simulink model "SpaceVectorPWM"  (R2018a)
settings: Solver=FixedStepDiscrete  StartTime=0.0  StopTime=0.2  FixedStep=1e-5  RelTol=1e-3
values from neighbouring files (symbols this model uses):
  A = 1    [SpaceVector.m]
  f_c = 5e4    (= 50000)    [PWM.m]    (also in SpaceVector.m = 50; SpwmTpwm.m = 50)
  f_s = 10000    [SpaceVector.m]    (also in SpaceVectorOnlyCode.m = 1000; SpwmTpwm.m)
undefined symbols (not defined in the file or in its folder): Vdc
libraries: simulink_extras x1, powerlib_meascontrol x1, simulink x1
settings Model: Creator=enes_  LastModifiedBy=enes_

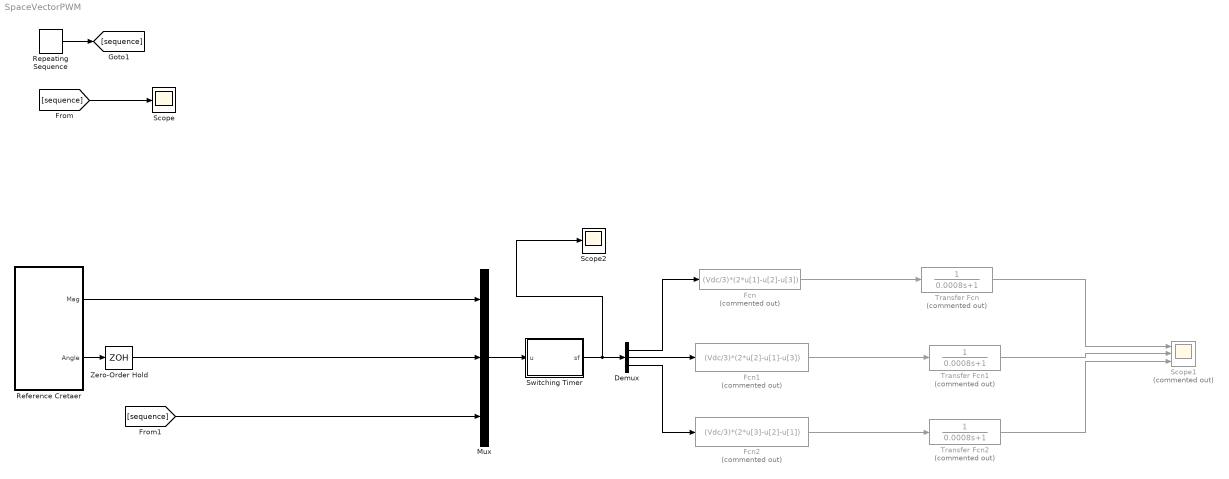
== system SpaceVectorPWM ==
  Demux : Demux  Outputs=3
  Fcn : Fcn  Commented=on  Expr=(Vdc/3)*(2*u[1]-u[2]-u[3])
  Fcn1 : Fcn  Commented=on  Expr=(Vdc/3)*(2*u[2]-u[1]-u[3])
  Fcn2 : Fcn  Commented=on  Expr=(Vdc/3)*(2*u[3]-u[2]-u[1])
  Mux : Mux  Inputs=3
  Reference Cretaer : Subsystem
  Repeating Sequence : simulink/Sources/Repeating Sequence  rep_seq_t=[0 1 2 3 4] /f_s  rep_seq_y=[-1 0 1 0 -1]
  Scope : Scope
  Scope1 : Scope  Commented=on  NumInputPorts=3
  Scope2 : Scope
  Switching Timer : MATLAB Function  TreatAsAtomicUnit=on
  Transfer Fcn : TransferFcn  Commented=on  Denominator=[0.0008 1]
  Transfer Fcn1 : TransferFcn  Commented=on  Denominator=[0.0008 1]
  Transfer Fcn2 : TransferFcn  Commented=on  Denominator=[0.0008 1]
  Zero-Order Hold : ZeroOrderHold  SampleTime=-1
  wires:
  [sequence] -> Scope/1
  Repeating Sequence/1 -> [sequence]
  Reference Cretaer/1("Mag ") -> Mux/1
  [sequence] -> Mux/3
  Reference Cretaer/2(Angle) -> Zero-Order Hold/1
  Zero-Order Hold/1 -> Mux/2
  Mux/1 -> Switching Timer/1(u)
  Switching Timer/1(sf) -> Demux/1, Scope2/1
  Fcn2/1 -> Transfer Fcn2/1
  Fcn1/1 -> Transfer Fcn1/1
  Fcn/1 -> Transfer Fcn/1
  Transfer Fcn/1 -> Scope1/1
  Transfer Fcn1/1 -> Scope1/2
  Transfer Fcn2/1 -> Scope1/3
  Demux/1 -> Fcn/1
  Demux/2 -> Fcn1/1
  Demux/3 -> Fcn2/1

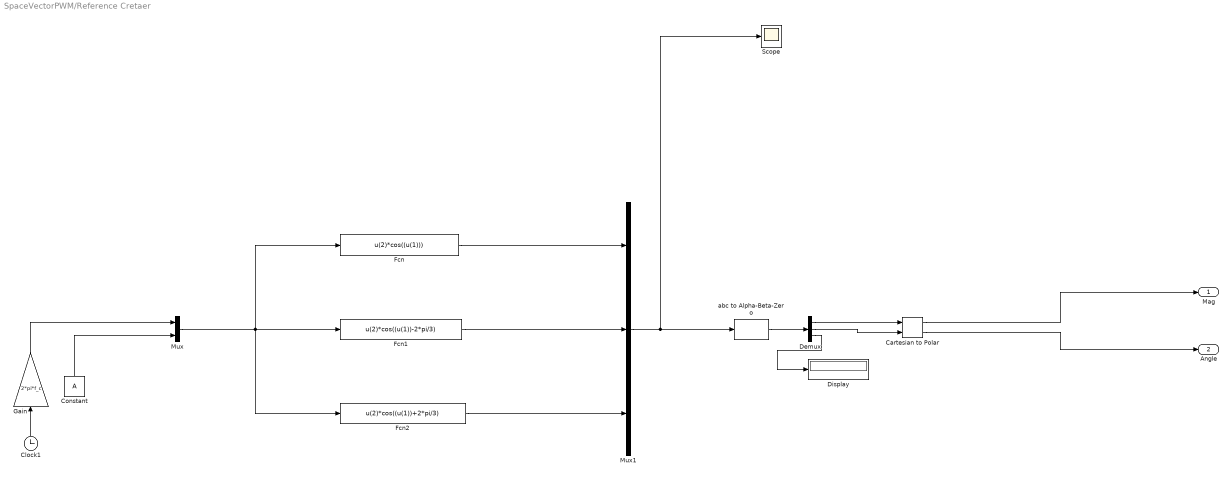
== system SpaceVectorPWM/Reference Cretaer ==
  Cartesian to Polar : simulink_extras/Transformations/Cartesian to Polar
      settings: SourceProductName=Simulink
  Clock1 : Clock
  Constant : Constant  Value=A
  Demux : Demux  Outputs=3
  Display : Display
  Fcn : Fcn  Expr=u(2)*cos((u(1)))
  Fcn1 : Fcn  Expr=u(2)*cos((u(1))-2*pi/3)
  Fcn2 : Fcn  Expr=u(2)*cos((u(1))+2*pi/3)
  Gain : Gain  Gain=2*pi*f_c
  Mux : Mux  Inputs=2
  Mux1 : Mux  Inputs=3
  Scope : Scope
  abc to Alpha-Beta-Zero : powerlib_meascontrol/Transformations/abc to Alpha-Beta-Zero
      settings: SourceProductName=Simscape Power Systems
  "Mag " : Outport
  Angle : Outport  Port=2
  wires:
  Mux/1 -> Fcn2/1, Fcn1/1, Fcn/1
  Constant/1 -> Mux/2
  Gain/1 -> Mux/1
  Mux1/1 -> abc to Alpha-Beta-Zero/1, Scope/1
  Fcn2/1 -> Mux1/3
  Fcn/1 -> Mux1/1
  Clock1/1 -> Gain/1
  Fcn1/1 -> Mux1/2
  abc to Alpha-Beta-Zero/1 -> Demux/1
  Demux/1 -> Cartesian to Polar/1
  Demux/2 -> Cartesian to Polar/2
  Cartesian to Polar/1 -> "Mag "/1
  Cartesian to Polar/2 -> Angle/1
  Demux/3 -> Display/1

== matlab function SpaceVectorPWM/Switching Timer ==
  data: u input; sf output
%Matlab Code to generate Switching functions
% Inputs are magnitude u1(:),angle u2(:)
% and ramp time signal for comparison u3(:)
function sf =SwitchingTimer(u)
ts=0.0002;vdc=1;peak_phase_max= vdc/sqrt(3);
x=u(2); y=u(3); mag=(u(1)/peak_phase_max) * ts;
%sector I
 if (x>=0) & (x<pi/3)
 ta = mag * sin(pi/3-x);tb = mag * sin(x);
 t0 =(ts-ta-tb);
t1=[t0/4 ta/2 tb/2 t0/2 tb/2 ta/2 t0/4];t1=cumsum(t1);
v1=[0 1 1 1 1 1 0];v2=[0 0 1 1 1 0 0];v3=[0 0 0 1 0 0 0];
 for j=1:7
 if(y<t1(j))
 break
 end
 end
 sa=v1(j);sb=v2(j);sc=v3(j);
end
% sector II
 if (x>=pi/3) & (x<2*pi/3)
 adv= x-pi/3;
tb = mag * sin(pi/3-adv);ta = mag * sin(adv);
t0 =(ts-ta-tb);
t1=[t0/4 ta/2 tb/2 t0/2 tb/2 ta/2 t0/4];t1=cumsum(t1);
v1=[0 0 1 1 1 0 0];v2=[0 1 1 1 1 1 0];v3=[0 0 0 1 0 0 0];
 for j=1:7
 if(y<t1(j))
 break
 end
 end
 sa=v1(j);sb=v2(j);sc=v3(j);
 end
%sector III
 if (x>=2*pi/3) & (x<pi)
 adv=x-2*pi/3;
ta = mag * sin(pi/3-adv);tb = mag * sin(adv);
 t0 =(ts-ta-tb);
t1=[t0/4 ta/2 tb/2 t0/2 tb/2 ta/2 t0/4];t1=cumsum(t1);
v1=[0 0 0 1 0 0 0];v2=[0 1 1 1 1 1 0];v3=[0 0 1 1 1 0 0];
 for j=1:7
 if(y<t1(j))
 break
 end
 end
 sa=v1(j);sb=v2(j);sc=v3(j);
end
%sector IV
 if (x>=-pi) & (x<-2*pi/3)
 adv = x + pi;
tb= mag * sin(pi/3 - adv);ta = mag * sin(adv);
 t0 =(ts-ta-tb);
t1=[t0/4 ta/2 tb/2 t0/2 tb/2 ta/2 t0/4];t1=cumsum(t1);
v1=[0 0 0 1 0 0 0];v2=[0 0 1 1 1 0 0];v3=[0 1 1 1 1 1 0];
 for j=1:7
 if(y<t1(j))
 break
 end
 end
 sa=v1(j);sb=v2(j);sc=v3(j);
end
% sector V
 if (x>=-2*pi/3) & (x<-pi/3)
 adv = x+2*pi/3;
ta = mag * sin(pi/3-adv);tb = mag * sin(adv);
 t0 =(ts-ta-tb);
t1=[t0/4 ta/2 tb/2 t0/2 tb/2 ta/2 t0/4];t1=cumsum(t1);
v1=[0 0 1 1 1 0 0];v2=[0 0 0 1 0 0 0];v3=[0 1 1 1 1 1 0];
 for j=1:7
 if(y<t1(j))
 break
 end
 end
 sa=v1(j);sb=v2(j);sc=v3(j);
end
%Sector VI
 if (x>=-pi/3) & (x<0)
 adv = x+pi/3;
tb = mag * sin(pi/3-adv);ta = mag * sin(adv);
 t0 =(ts-ta-tb);
t1=[t0/4 ta/2 tb/2 t0/2 tb/2 ta/2 t0/4];t1=cumsum(t1);
v1=[0 1 1 1 1 1 0];v2=[0 0 0 1 0 0 0];v3=[0 0 1 1 1 0 0];
 for j=1:7
 if(y<t1(j))
 break
 end
 end
 sa=v1(j);sb=v2(j);sc=v3(j);
end
 sf=[sa, sb, sc];
